simulink model "lqr_cascada"  (R2025b)
settings: Solver=VariableStepAuto  StartTime=0.0  StopTime=10  RelTol=1e-3
undefined symbols (not defined in the file or in its folder): Ka, Ki, N
settings Model: Creator=rel  LastModifiedBy=rel

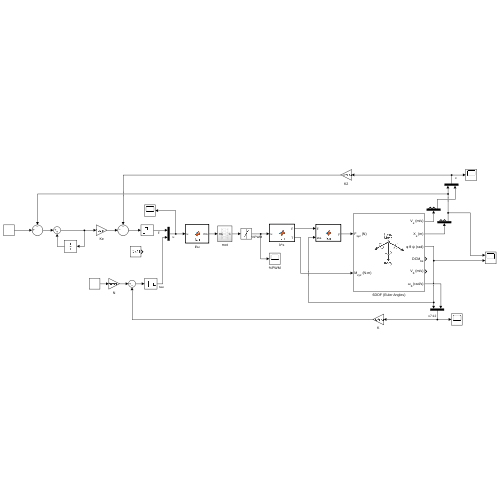
[thumbnail: Simulink's stored preview of the top-level diagram]
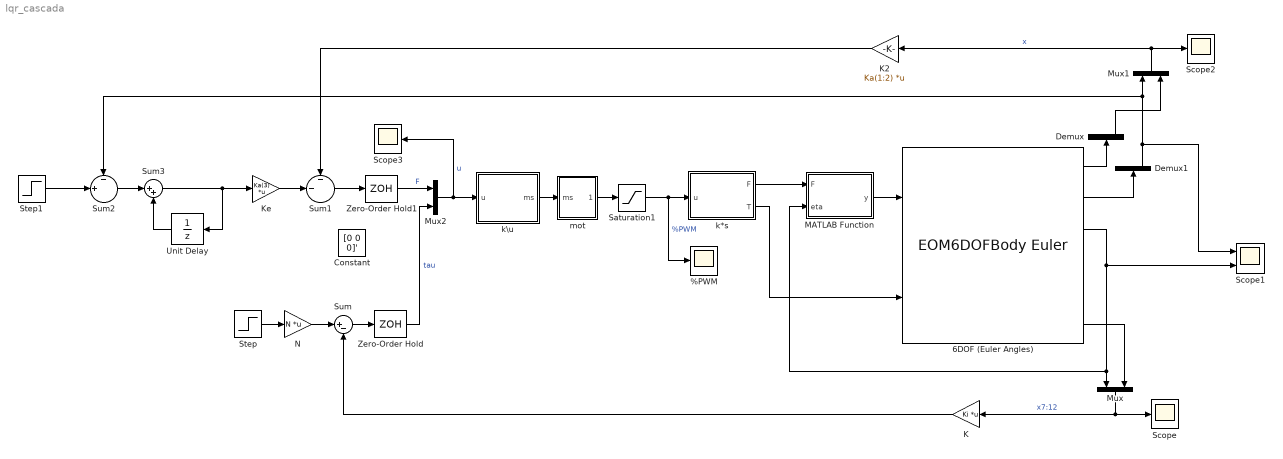
== system lqr_cascada ==
  %PWM : Scope
      settings: ActiveDisplayYMinimum=-1  ActiveDisplayYMaximum=1  DataLoggingVariableName=ScopeData4
  6DOF (Euler Angles) : EOM6DOFBodyEuler  mass_0=1.6  inertia=diag([0.021915027 0.022124548 0.042349865])
  Constant : Constant  Value=[0 0 0]'
  Demux : Demux  Outputs=3
  Demux1 : Demux  Outputs=3
  K : Gain  Gain=Ki  Multiplication=Matrix(K*u) (u vector)
  K2 : Gain  Gain=Ka(1:2)  Multiplication=Matrix(K*u) (u vector)
  Ke : Gain  Gain=Ka(3)  Multiplication=Matrix(K*u) (u vector)
  MATLAB Function : MATLAB Function  TreatAsAtomicUnit=on
  Mux : Mux  Inputs=2
  Mux1 : Mux  Inputs=2
  Mux2 : Mux  Inputs=2
  N : Gain  Gain=N  Multiplication=Matrix(K*u) (u vector)
  Saturation1 : Saturate  UpperLimit=1  LowerLimit=0
  Scope : Scope
      settings: ActiveDisplayYMinimum=-1  ActiveDisplayYMaximum=1
  Scope1 : Scope  NumInputPorts=2
      settings: ActiveDisplayYMinimum=-0.60964636028716812  ActiveDisplayYMaximum=1.2577680656974948
  Scope2 : Scope
      settings: ActiveDisplayYMinimum=-1.0699839344999873  ActiveDisplayYMaximum=2.6160785638185868  DataLoggingVariableName=ScopeData2
  Scope3 : Scope
      settings: ActiveDisplayYMinimum=-17.234606604861909  ActiveDisplayYMaximum=28.714896837749958  DataLoggingVariableName=ScopeData3
  Step : Step  Time=[5 5.5 5.8]  Before=[0 0 0]  After=deg2rad([20 20 20])  SampleTime=0
  Step1 : Step  SampleTime=0
  Sum : Sum  Inputs=|+-
  Sum1 : Sum  Inputs=-|-||
  Sum2 : Sum  Inputs=-|+||
  Sum3 : Sum  Inputs=|++
  Unit Delay : UnitDelay  SampleTime=1/100  HasFrameUpgradeWarning=on
  Zero-Order Hold : ZeroOrderHold  SampleTime=1/510
  Zero-Order Hold1 : ZeroOrderHold  SampleTime=1/100
  k*s : MATLAB Function  TreatAsAtomicUnit=on
  k\u : MATLAB Function  TreatAsAtomicUnit=on
  mot : Subsystem
  wires:
  Step/1 -> N/1
  N/1 -> Sum/1
  6DOF (Euler Angles)/3 -> MATLAB Function/2(eta), Mux/1, Scope1/2
  6DOF (Euler Angles)/6 -> Mux/2
  Mux/1 -> K/1, Scope/1  "x7:12"
  Sum/1 -> Zero-Order Hold/1
  K/1 -> Sum/2
  mot/1(Out1) -> Saturation1/1
  Saturation1/1 -> %PWM/1, k*s/1(u)  "%PWM"
  k\u/1(ms) -> mot/1(ms)
  MATLAB Function/1(y) -> 6DOF (Euler Angles)/1
  6DOF (Euler Angles)/2 -> Demux1/1
  6DOF (Euler Angles)/1 -> Demux/1
  Demux/3 -> Mux1/2
  Mux1/1 -> K2/1, Scope2/1  "x"
  K2/1 -> Sum1/1
  Zero-Order Hold1/1 -> Mux2/1  "F"
  Mux2/1 -> Scope3/1, k\u/1(u)  "u"
  Sum1/1 -> Zero-Order Hold1/1
  Step1/1 -> Sum2/2
  k*s/1(F) -> MATLAB Function/1(F)
  Demux1/3 -> Sum2/1, Mux1/1, Scope1/1
  k*s/2(T) -> 6DOF (Euler Angles)/2
  Sum2/1 -> Sum3/1
  Unit Delay/1 -> Sum3/2
  Ke/1 -> Sum1/2
  Sum3/1 -> Unit Delay/1, Ke/1
  Zero-Order Hold/1 -> Mux2/2  "tau"

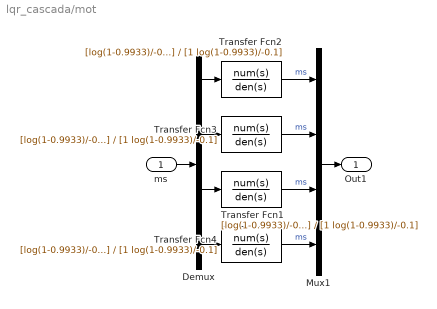
== system lqr_cascada/mot ==
  ms : Inport
  Demux : Demux
  Mux1 : Mux
  Transfer Fcn{1..4} (4 alike) : TransferFcn  Numerator=[log(1-0.9933)/-0.1]  Denominator=[1 log(1-0.9933)/-0.1]
  Out1 : Outport
  wires:
  Transfer Fcn3/1 -> Mux1/2  "ms"
  Transfer Fcn1/1 -> Mux1/3  "ms"
  Demux/3 -> Transfer Fcn1/1
  Transfer Fcn4/1 -> Mux1/4  "ms"
  Demux/4 -> Transfer Fcn4/1
  Mux1/1 -> Out1/1
  Transfer Fcn2/1 -> Mux1/1  "ms"
  Demux/2 -> Transfer Fcn3/1
  Demux/1 -> Transfer Fcn2/1
  ms/1 -> Demux/1

== matlab function lqr_cascada/k\u ==
  data: u input; ms output
function ms = fcn(u)
% L = 0.0080;
% kF = 0.1600*9.81;
% kM = 0.0086;
L = 0.268554;
kF = 7.965;
kM = 0.2;
A = [kF kF kF kF; -L*kF -L*kF L*kF L*kF; L*kF -L*kF -L*kF L*kF; -kM kM -kM kM];
ms = A\[u(1); u(2:end)];

== matlab function lqr_cascada/MATLAB Function ==
  data: F input; y output; eta input
function y = fcn(F, eta)
phi = eta(1);
theta = eta(2);
psi = eta(3);
y = [0;0;-1.6*9.81] + [sin(theta)*cos(psi) + sin(phi)*cos(theta)*sin(psi); ...
                    sin(theta)*sin(psi) - sin(phi)*cos(theta)*cos(psi); ...
                    cos(phi)*cos(theta)]*F;

== matlab function lqr_cascada/k*s ==
  data: u input; F output; T output
function [F, T] = fcn(u)
% L = 0.0080;
% kF = 0.1600*9.81;
% kM = 0.0086;
L = 0.268554;
kF = 7.965;
kM = 0.2;
A = [kF kF kF kF; -L*kF -L*kF L*kF L*kF; L*kF -L*kF -L*kF L*kF; -kM kM -kM kM];
y = A*u;
F = y(1);
T = y(2:end);
